simulink model "model21"  (R2021a)
settings: Solver=VariableStepAuto  StartTime=0.0  StopTime=60  RelTol=1e-3
values from neighbouring files (symbols this model uses):
  Ax = 0.8    [model2.m]
  Ay = 0.8    [model2.m]
  Az = 0.4    [model2.m]
  b = 3.59*10^-5    (= 3.59e-05)    [model2.m]
  d = 2.0810*10^-6    (= 2.081e-06)    [model2.m]
  g = 9.81    [model2.m]
  Ix = 0.04439    [model2.m]
  Iy = 0.04439    [model2.m]
  Iz = 0.019    [model2.m]
  J = 0.045    [model2.m]
  l = 0.24    [model2.m]
  m = 0.99285    [model2.m]
undefined symbols (not defined in the file or in its folder): sigbuilder_block
libraries: pid_lib x4
settings Model: Creator=hp  LastModifiedBy=ANUDEEP
settings SolverCC: AlgebraicLoopSolver=TrustRegion
settings DebuggingCC: SFMachineParentedDataDiag=warning

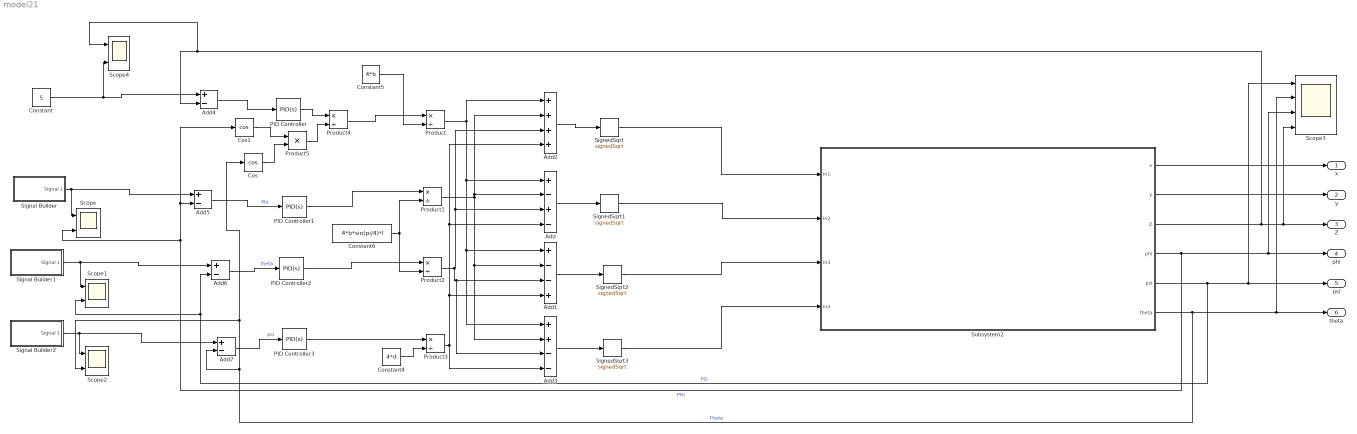
== system model21 ==
  Add : Sum  Inputs=+-+-
  Add1 : Sum  Inputs=+--+
  Add2 : Sum  Inputs=++++
  Add3 : Sum  Inputs=++--
  Add{4..7} (4 alike) : Sum  Inputs=+-
  Constant : Constant  Value=5
  Constant4 : Constant  Value=4*d
  Constant5 : Constant  Value=4*b
  Constant6 : Constant  Value=4*b*sin(pi/4)*l
  Cos : Trigonometry  Operator=cos
  Cos1 : Trigonometry  Operator=cos
  PID Controller : pid_lib/PID Controller  Controller=PID  Form=Parallel  TimeDomain=Continuous-time  UseExternalTs=off  SampleTime=-1  IntegratorMethod=Forward Euler  FilterMethod=Forward Euler  ControllerParametersSource=internal  P=4.3  I=4.5  D=2.05  UseFilter=on  N=100  TunerSelectOption=Transfer Function Based (PID Tuner App)  InitialConditionSource=internal  InitialConditionForIntegrator=0  InitialConditionForFilter=0  DifferentiatorICPrevScaledInput=0  ExternalReset=none  TrackingMode=off  Kt=1  LimitOutput=off  SatLimitsSource=internal  UpperSaturationLimit=inf  LowerSaturationLimit=-inf  LinearizeAsGain=on  AntiWindupMode=none  Kb=1  POutMin=[]  POutMax=[]  IOutMin=[]  IOutMax=[]  DOutMin=[]  DOutMax=[]  NOutMin=[]  NOutMax=[]  SumOutMin=[]  SumOutMax=[]  SaturationOutMin=[]  SaturationOutMax=[]  PParamMin=[]  PParamMax=[]  IParamMin=[]  IParamMax=[]  DParamMin=[]  DParamMax=[]  NParamMin=[]  NParamMax=[]  KbParamMin=[]  KbParamMax=[]  KtParamMin=[]  KtParamMax=[]  KbOutMin=[]  KbOutMax=[]  KtOutMin=[]  KtOutMax=[]  IntegratorOutMin=[]  IntegratorOutMax=[]  FilterOutMin=[]  FilterOutMax=[]  SumI1OutMin=[]  SumI1OutMax=[]  SumI2OutMin=[]  SumI2OutMax=[]  SumI3OutMin=[]  SumI3OutMax=[]  SumI4OutMin=[]  SumI4OutMax=[]  SumDOutMin=[]  SumDOutMax=[]  DifferentiatorOutMin=[]  DifferentiatorOutMax=[]  FilterDiffOutCoefMin=[]  FilterDiffOutCoefMax=[]  ReciprocalOutMin=[]  ReciprocalOutMax=[]  SumDenOutMin=[]  SumDenOutMax=[]  SumNumOutMin=[]  SumNumOutMax=[]  DivideOutMin=[]  DivideOutMax=[]  UdiffTsProdOutMin=[]  UdiffTsProdOutMax=[]  NTsProdOutMin=[]  NTsProdOutMax=[]  UintegralTsProdOutMin=[]  UintegralTsProdOutMax=[]  UngainTsProdOutMin=[]  UngainTsProdOutMax=[]  IntegratorContinuousStateAttributes=''  IntegratorStateMustResolveToSignalObject=off  IntegratorRTWStateStorageClass=Auto  FilterContinuousStateAttributes=''  FilterStateMustResolveToSignalObject=off  FilterRTWStateStorageClass=Auto  ParallelPVariant=InternalParameters  IdealPVariant=Disabled  IVariant=InternalParameters  DVariant=InternalParameters  IntegratorVariant=Continuous  SatVariant=Disabled  AWVariant=Passthrough  PCopyVariant=Disabled  TRVariant=Disabled  FdbkBlocksVariant=Forward  IdealPFdbkVariant=Disabled  SatFdbkVariant=Disabled  DerivativeFilterVariant=ContFilter  NVariant=InternalParameters  NCopyVariant=Disabled  FilterICVariant=InternalICsFilter  IntegratorICVariant=InternalICs  ExternalResetVariant=Disabled  TRSumVariant=Passthrough  SumFdbkVariant=Disabled  SumVariant=Sum_PID  TsampFilterVariant=InternalTs  TsampNgainVariant=Passthrough  TsampIntegralVariant=Passthrough  ExternalSaturationOutDataTypeStr=Inherit: Same as second input
  PID Controller1 : pid_lib/PID Controller  Controller=PID  Form=Parallel  TimeDomain=Continuous-time  UseExternalTs=off  SampleTime=-1  IntegratorMethod=Forward Euler  FilterMethod=Forward Euler  ControllerParametersSource=internal  P=0.262692793721386  I=0.0679116483715347  D=0.252983550233798  UseFilter=on  N=657.62885892053  TunerSelectOption=Transfer Function Based (PID Tuner App)  InitialConditionSource=internal  InitialConditionForIntegrator=0  InitialConditionForFilter=0  DifferentiatorICPrevScaledInput=0  ExternalReset=none  TrackingMode=off  Kt=1  LimitOutput=off  SatLimitsSource=internal  UpperSaturationLimit=inf  LowerSaturationLimit=-inf  LinearizeAsGain=on  AntiWindupMode=none  Kb=1  POutMin=[]  POutMax=[]  IOutMin=[]  IOutMax=[]  DOutMin=[]  DOutMax=[]  NOutMin=[]  NOutMax=[]  SumOutMin=[]  SumOutMax=[]  SaturationOutMin=[]  SaturationOutMax=[]  PParamMin=[]  PParamMax=[]  IParamMin=[]  IParamMax=[]  DParamMin=[]  DParamMax=[]  NParamMin=[]  NParamMax=[]  KbParamMin=[]  KbParamMax=[]  KtParamMin=[]  KtParamMax=[]  KbOutMin=[]  KbOutMax=[]  KtOutMin=[]  KtOutMax=[]  IntegratorOutMin=[]  IntegratorOutMax=[]  FilterOutMin=[]  FilterOutMax=[]  SumI1OutMin=[]  SumI1OutMax=[]  SumI2OutMin=[]  SumI2OutMax=[]  SumI3OutMin=[]  SumI3OutMax=[]  SumI4OutMin=[]  SumI4OutMax=[]  SumDOutMin=[]  SumDOutMax=[]  DifferentiatorOutMin=[]  DifferentiatorOutMax=[]  FilterDiffOutCoefMin=[]  FilterDiffOutCoefMax=[]  ReciprocalOutMin=[]  ReciprocalOutMax=[]  SumDenOutMin=[]  SumDenOutMax=[]  SumNumOutMin=[]  SumNumOutMax=[]  DivideOutMin=[]  DivideOutMax=[]  UdiffTsProdOutMin=[]  UdiffTsProdOutMax=[]  NTsProdOutMin=[]  NTsProdOutMax=[]  UintegralTsProdOutMin=[]  UintegralTsProdOutMax=[]  UngainTsProdOutMin=[]  UngainTsProdOutMax=[]  IntegratorContinuousStateAttributes=''  IntegratorStateMustResolveToSignalObject=off  IntegratorRTWStateStorageClass=Auto  FilterContinuousStateAttributes=''  FilterStateMustResolveToSignalObject=off  FilterRTWStateStorageClass=Auto  ParallelPVariant=InternalParameters  IdealPVariant=Disabled  IVariant=InternalParameters  DVariant=InternalParameters  IntegratorVariant=Continuous  SatVariant=Disabled  AWVariant=Passthrough  PCopyVariant=Disabled  TRVariant=Disabled  FdbkBlocksVariant=Forward  IdealPFdbkVariant=Disabled  SatFdbkVariant=Disabled  DerivativeFilterVariant=ContFilter  NVariant=InternalParameters  NCopyVariant=Disabled  FilterICVariant=InternalICsFilter  IntegratorICVariant=InternalICs  ExternalResetVariant=Disabled  TRSumVariant=Passthrough  SumFdbkVariant=Disabled  SumVariant=Sum_PID  TsampFilterVariant=InternalTs  TsampNgainVariant=Passthrough  TsampIntegralVariant=Passthrough  ExternalSaturationOutDataTypeStr=Inherit: Same as second input
  PID Controller2 : pid_lib/PID Controller  Controller=PID  Form=Parallel  TimeDomain=Continuous-time  UseExternalTs=off  SampleTime=-1  IntegratorMethod=Forward Euler  FilterMethod=Forward Euler  ControllerParametersSource=internal  P=0.314077810197869  I=0.074408762657649  D=0.304896946822323  UseFilter=on  N=790.643788258186  TunerSelectOption=Transfer Function Based (PID Tuner App)  InitialConditionSource=internal  InitialConditionForIntegrator=0  InitialConditionForFilter=0  DifferentiatorICPrevScaledInput=0  ExternalReset=none  TrackingMode=off  Kt=1  LimitOutput=off  SatLimitsSource=internal  UpperSaturationLimit=inf  LowerSaturationLimit=-inf  LinearizeAsGain=on  AntiWindupMode=none  Kb=1  POutMin=[]  POutMax=[]  IOutMin=[]  IOutMax=[]  DOutMin=[]  DOutMax=[]  NOutMin=[]  NOutMax=[]  SumOutMin=[]  SumOutMax=[]  SaturationOutMin=[]  SaturationOutMax=[]  PParamMin=[]  PParamMax=[]  IParamMin=[]  IParamMax=[]  DParamMin=[]  DParamMax=[]  NParamMin=[]  NParamMax=[]  KbParamMin=[]  KbParamMax=[]  KtParamMin=[]  KtParamMax=[]  KbOutMin=[]  KbOutMax=[]  KtOutMin=[]  KtOutMax=[]  IntegratorOutMin=[]  IntegratorOutMax=[]  FilterOutMin=[]  FilterOutMax=[]  SumI1OutMin=[]  SumI1OutMax=[]  SumI2OutMin=[]  SumI2OutMax=[]  SumI3OutMin=[]  SumI3OutMax=[]  SumI4OutMin=[]  SumI4OutMax=[]  SumDOutMin=[]  SumDOutMax=[]  DifferentiatorOutMin=[]  DifferentiatorOutMax=[]  FilterDiffOutCoefMin=[]  FilterDiffOutCoefMax=[]  ReciprocalOutMin=[]  ReciprocalOutMax=[]  SumDenOutMin=[]  SumDenOutMax=[]  SumNumOutMin=[]  SumNumOutMax=[]  DivideOutMin=[]  DivideOutMax=[]  UdiffTsProdOutMin=[]  UdiffTsProdOutMax=[]  NTsProdOutMin=[]  NTsProdOutMax=[]  UintegralTsProdOutMin=[]  UintegralTsProdOutMax=[]  UngainTsProdOutMin=[]  UngainTsProdOutMax=[]  IntegratorContinuousStateAttributes=''  IntegratorStateMustResolveToSignalObject=off  IntegratorRTWStateStorageClass=Auto  FilterContinuousStateAttributes=''  FilterStateMustResolveToSignalObject=off  FilterRTWStateStorageClass=Auto  ParallelPVariant=InternalParameters  IdealPVariant=Disabled  IVariant=InternalParameters  DVariant=InternalParameters  IntegratorVariant=Continuous  SatVariant=Disabled  AWVariant=Passthrough  PCopyVariant=Disabled  TRVariant=Disabled  FdbkBlocksVariant=Forward  IdealPFdbkVariant=Disabled  SatFdbkVariant=Disabled  DerivativeFilterVariant=ContFilter  NVariant=InternalParameters  NCopyVariant=Disabled  FilterICVariant=InternalICsFilter  IntegratorICVariant=InternalICs  ExternalResetVariant=Disabled  TRSumVariant=Passthrough  SumFdbkVariant=Disabled  SumVariant=Sum_PID  TsampFilterVariant=InternalTs  TsampNgainVariant=Passthrough  TsampIntegralVariant=Passthrough  ExternalSaturationOutDataTypeStr=Inherit: Same as second input
  PID Controller3 : pid_lib/PID Controller  Controller=PID  Form=Parallel  TimeDomain=Continuous-time  UseExternalTs=off  SampleTime=-1  IntegratorMethod=Forward Euler  FilterMethod=Forward Euler  ControllerParametersSource=internal  P=0.003528  I=0.0001652  D=0.0185  UseFilter=on  N=5.454  TunerSelectOption=Transfer Function Based (PID Tuner App)  InitialConditionSource=internal  InitialConditionForIntegrator=0  InitialConditionForFilter=0  DifferentiatorICPrevScaledInput=0  ExternalReset=none  TrackingMode=off  Kt=1  LimitOutput=off  SatLimitsSource=internal  UpperSaturationLimit=inf  LowerSaturationLimit=-inf  LinearizeAsGain=on  AntiWindupMode=none  Kb=1  POutMin=[]  POutMax=[]  IOutMin=[]  IOutMax=[]  DOutMin=[]  DOutMax=[]  NOutMin=[]  NOutMax=[]  SumOutMin=[]  SumOutMax=[]  SaturationOutMin=[]  SaturationOutMax=[]  PParamMin=[]  PParamMax=[]  IParamMin=[]  IParamMax=[]  DParamMin=[]  DParamMax=[]  NParamMin=[]  NParamMax=[]  KbParamMin=[]  KbParamMax=[]  KtParamMin=[]  KtParamMax=[]  KbOutMin=[]  KbOutMax=[]  KtOutMin=[]  KtOutMax=[]  IntegratorOutMin=[]  IntegratorOutMax=[]  FilterOutMin=[]  FilterOutMax=[]  SumI1OutMin=[]  SumI1OutMax=[]  SumI2OutMin=[]  SumI2OutMax=[]  SumI3OutMin=[]  SumI3OutMax=[]  SumI4OutMin=[]  SumI4OutMax=[]  SumDOutMin=[]  SumDOutMax=[]  DifferentiatorOutMin=[]  DifferentiatorOutMax=[]  FilterDiffOutCoefMin=[]  FilterDiffOutCoefMax=[]  ReciprocalOutMin=[]  ReciprocalOutMax=[]  SumDenOutMin=[]  SumDenOutMax=[]  SumNumOutMin=[]  SumNumOutMax=[]  DivideOutMin=[]  DivideOutMax=[]  UdiffTsProdOutMin=[]  UdiffTsProdOutMax=[]  NTsProdOutMin=[]  NTsProdOutMax=[]  UintegralTsProdOutMin=[]  UintegralTsProdOutMax=[]  UngainTsProdOutMin=[]  UngainTsProdOutMax=[]  IntegratorContinuousStateAttributes=''  IntegratorStateMustResolveToSignalObject=off  IntegratorRTWStateStorageClass=Auto  FilterContinuousStateAttributes=''  FilterStateMustResolveToSignalObject=off  FilterRTWStateStorageClass=Auto  ParallelPVariant=InternalParameters  IdealPVariant=Disabled  IVariant=InternalParameters  DVariant=InternalParameters  IntegratorVariant=Continuous  SatVariant=Disabled  AWVariant=Passthrough  PCopyVariant=Disabled  TRVariant=Disabled  FdbkBlocksVariant=Forward  IdealPFdbkVariant=Disabled  SatFdbkVariant=Disabled  DerivativeFilterVariant=ContFilter  NVariant=InternalParameters  NCopyVariant=Disabled  FilterICVariant=InternalICsFilter  IntegratorICVariant=InternalICs  ExternalResetVariant=Disabled  TRSumVariant=Passthrough  SumFdbkVariant=Disabled  SumVariant=Sum_PID  TsampFilterVariant=InternalTs  TsampNgainVariant=Passthrough  TsampIntegralVariant=Passthrough  ExternalSaturationOutDataTypeStr=Inherit: Same as second input
  Product{,1..4} (5 alike) : Product  Inputs=*/
  Product5 : Product
  Scope{,1..2,4} (4 alike) : Scope  NumInputPorts=2
  Scope3 : Scope  NumInputPorts=4
  Signal Builder : Subsystem  Tag=STV Subsys  LoadFcn=sigbuilder_block('load');  StartFcn=sigbuilder_block('start');  StopFcn=sigbuilder_block('stop');  ClipboardFcn=sigbuilder_block('clipboard');  mask(Sigbuilder block){tuvar=[0:10]}
      mask help: Simulink:masks:SigbuilderBlock_MD
      mask init:
      | if ~strcmp(get_param(bdroot(gcbh),'SimulationStatus'),'stopped') tuvar = sigbuilder_block('maskInit'); end
      settings: CopyFcn=sigbuilder_block('copy');  DeleteFcn=sigbuilder_block('delete');  ModelCloseFcn=sigbuilder_block('modelClose');  PreSaveFcn=sigbuilder_block('preSave');  PauseFcn=sigbuilder_block('pause');  ContinueFcn=sigbuilder_block('continue');  NameChangeFcn=sigbuilder_block('namechange');  OpenFcn=sigbuilder_block('open',[367.8 129.6 550.8 400.2 ]);  CloseFcn=sigbuilder_block('close');
      mask Display: plot(0, 0, 100, 100,[2, 2, 32, 32, 2], [68, 8, 8, 68, 68],[32, 2], [38, 38], [32, 19, 2],[53, 60, 44], [32, 17, 17, 2],[16, 16, 31, 31]);txt = getActiveGroup(gcbh);text(2, 100, txt,'verticalAlignment', 'top');
  Signal Builder1 : Subsystem  Tag=STV Subsys  LoadFcn=sigbuilder_block('load');  StartFcn=sigbuilder_block('start');  StopFcn=sigbuilder_block('stop');  ClipboardFcn=sigbuilder_block('clipboard');  mask(Sigbuilder block){tuvar=[0:10]}
      mask help: Simulink:masks:SigbuilderBlock_MD
      mask init:
      | if ~strcmp(get_param(bdroot(gcbh),'SimulationStatus'),'stopped') tuvar = sigbuilder_block('maskInit'); end
      settings: CopyFcn=sigbuilder_block('copy');  DeleteFcn=sigbuilder_block('delete');  ModelCloseFcn=sigbuilder_block('modelClose');  PreSaveFcn=sigbuilder_block('preSave');  PauseFcn=sigbuilder_block('pause');  ContinueFcn=sigbuilder_block('continue');  NameChangeFcn=sigbuilder_block('namechange');  OpenFcn=sigbuilder_block('open',[367.8 129.6 550.8 400.2 ]);  CloseFcn=sigbuilder_block('close');
      mask Display: plot(0, 0, 100, 100,[2, 2, 32, 32, 2], [68, 8, 8, 68, 68],[32, 2], [38, 38], [32, 19, 2],[53, 60, 44], [32, 17, 17, 2],[16, 16, 31, 31]);txt = getActiveGroup(gcbh);text(2, 100, txt,'verticalAlignment', 'top');
  Signal Builder2 : Subsystem  Tag=STV Subsys  LoadFcn=sigbuilder_block('load');  StartFcn=sigbuilder_block('start');  StopFcn=sigbuilder_block('stop');  ClipboardFcn=sigbuilder_block('clipboard');  mask(Sigbuilder block){tuvar=[0:10]}
      mask help: Simulink:masks:SigbuilderBlock_MD
      mask init:
      | if ~strcmp(get_param(bdroot(gcbh),'SimulationStatus'),'stopped') tuvar = sigbuilder_block('maskInit'); end
      settings: CopyFcn=sigbuilder_block('copy');  DeleteFcn=sigbuilder_block('delete');  ModelCloseFcn=sigbuilder_block('modelClose');  PreSaveFcn=sigbuilder_block('preSave');  PauseFcn=sigbuilder_block('pause');  ContinueFcn=sigbuilder_block('continue');  NameChangeFcn=sigbuilder_block('namechange');  OpenFcn=sigbuilder_block('open',[345.6 111.6 550.8 400.2 ]);  CloseFcn=sigbuilder_block('close');
      mask Display: plot(0, 0, 100, 100,[2, 2, 32, 32, 2], [68, 8, 8, 68, 68],[32, 2], [38, 38], [32, 19, 2],[53, 60, 44], [32, 17, 17, 2],[16, 16, 31, 31]);txt = getActiveGroup(gcbh);text(2, 100, txt,'verticalAlignment', 'top');
  SignedSqrt{,1..3} (4 alike) : Sqrt  Operator=signedSqrt  OutputSignalType=real  IntermediateResultsDataTypeStr=single  SaturateOnIntegerOverflow=on
  Subsystem2 : Subsystem
  x : Outport
  y : Outport  Port=2
  Z : Outport  Port=3
  phi : Outport  Port=4
  psi : Outport  Port=5
  theta : Outport  Port=6
  wires:
  Product/1 -> Add1/1, Add3/1, Add/1, Add2/1
  Product1/1 -> Add/2, Add2/2, Add1/2, Add3/2
  Product2/1 -> Add3/3, Add1/3, Add/3, Add2/3
  Product3/1 -> Add1/4, Add/4, Add2/4, Add3/4
  Constant4/1 -> Product3/2
  Constant5/1 -> Product/2
  Constant6/1 -> Product1/2, Product2/2
  Product4/1 -> Product/1
  PID Controller/1 -> Product4/1
  Product5/1 -> Product4/2
  Cos/1 -> Product5/2
  Cos1/1 -> Product5/1
  Add4/1 -> PID Controller/1
  PID Controller1/1 -> Product1/1
  PID Controller2/1 -> Product2/1
  PID Controller3/1 -> Product3/1
  Add2/1 -> SignedSqrt/1
  Add/1 -> SignedSqrt1/1
  Add1/1 -> SignedSqrt2/1
  Add3/1 -> SignedSqrt3/1
  Subsystem2/1(x) -> x/1
  Subsystem2/2(y) -> y/1
  Subsystem2/3(Z) -> Scope4/1, Add4/2, Scope3/4, Z/1
  Subsystem2/4(phi) -> Scope/2, Cos1/1, Add5/2, Scope3/3, phi/1  "PHI"
  Subsystem2/5(psi) -> Add6/2, Scope1/2, Scope3/1, psi/1  "PSI"
  Subsystem2/6(theta) -> Add7/2, Scope2/2, Cos/1, Scope3/2, theta/1  "Theta"
  Constant/1 -> Scope4/2, Add4/1
  Signal Builder/1(Signal 1) -> Scope/1, Add5/1
  Signal Builder1/1(Signal 1) -> Scope1/1, Add6/1
  Signal Builder2/1(Signal 1) -> Scope2/1, Add7/1
  Add7/1 -> PID Controller3/1  "psi"
  Add6/1 -> PID Controller2/1  "theta"
  Add5/1 -> PID Controller1/1  "Phi"
  SignedSqrt/1 -> Subsystem2/1(In1)
  SignedSqrt1/1 -> Subsystem2/2(In2)
  SignedSqrt2/1 -> Subsystem2/3(In3)
  SignedSqrt3/1 -> Subsystem2/4(In4)

== system model21/Signal Builder ==
  Demux : Demux  Tag=STV Demux  Outputs=1
      settings: DisplayOption=none
  FromWs : FromWorkspace  Tag=STV FromWs  VariableName=tuvar
      SigBuilderData=|
      | common.afterFinalStr = 'Extrapolate'
      | common.sampleTime = 0
      | dataSet.timeRange = [0 60]
      | dataSet.name = 'Group 1'
      | sbobj.Groups.Name = 'Group 1'
      | sbobj.Groups.Signals.Name = 'Signal 1'
      | sbobj.Groups.Signals.XData = [0 10 10 20 20 50 50 60]
      | sbobj.Groups.Signals.YData = [0 0 0.2 0.2 0 0 0.2 0.2]
      | sbobj.Groups.TimeRange = [0 60]
  Signal 1 : Outport  Tag=STV Outport
  wires:
  Demux/1 -> Signal 1/1
  FromWs/1 -> Demux/1

== system model21/Signal Builder1 ==
  Demux : Demux  Tag=STV Demux  Outputs=1
      settings: DisplayOption=none
  FromWs : FromWorkspace  Tag=STV FromWs  VariableName=tuvar
      SigBuilderData=|
      | common.afterFinalStr = 'Extrapolate'
      | common.sampleTime = 0
      | dataSet.timeRange = [0 60]
      | dataSet.name = 'Group 1'
      | sbobj.Groups.Name = 'Group 1'
      | sbobj.Groups.Signals.Name = 'Signal 1'
      | sbobj.Groups.Signals.XData = [0 30 30 40 40 60]
      | sbobj.Groups.Signals.YData = [0 0 0.2 0.2 0 0]
      | sbobj.Groups.TimeRange = [0 60]
  Signal 1 : Outport  Tag=STV Outport
  wires:
  Demux/1 -> Signal 1/1
  FromWs/1 -> Demux/1

== system model21/Signal Builder2 ==
  Demux : Demux  Tag=STV Demux  Outputs=1
      settings: DisplayOption=none
  FromWs : FromWorkspace  Tag=STV FromWs  VariableName=tuvar
      SigBuilderData=|
      | common.afterFinalStr = 'Extrapolate'
      | common.sampleTime = 0
      | dataSet.timeRange = [0 60]
      | dataSet.name = 'Group 1'
      | sbobj.Groups.Name = 'Group 1'
      | sbobj.Groups.Signals.Name = 'Signal 1'
      | sbobj.Groups.Signals.XData = [0 5 5 10 10 50 60]
      | sbobj.Groups.Signals.YData = [0 0 0.5 0.5 0 0 0]
      | sbobj.Groups.TimeRange = [0 60]
  Signal 1 : Outport  Tag=STV Outport
  wires:
  Demux/1 -> Signal 1/1
  FromWs/1 -> Demux/1

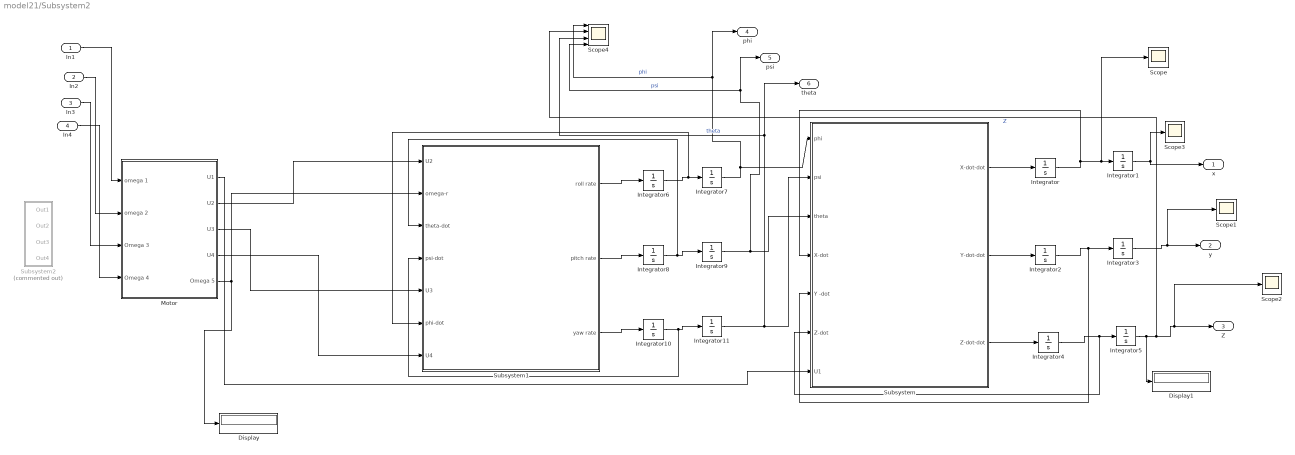
== system model21/Subsystem2 ==
  In1 : Inport
  In2 : Inport  Port=2
  In3 : Inport  Port=3
  In4 : Inport  Port=4
  Display : Display
  Display1 : Display
  Integrator{,1,3..4,6,8,10} (7 alike) : Integrator
  Integrator11 : Integrator  WrapState=on
  Integrator2 : Integrator  LimitOutput=on
  Integrator5 : Integrator  LimitOutput=on  LowerSaturationLimit=0
  Integrator7 : Integrator  WrapState=on
  Integrator9 : Integrator  WrapState=on
  Motor : Subsystem
  Scope{,1..3} (4 alike) : Scope
  Scope4 : Scope  NumInputPorts=4
  Subsystem : Subsystem
  Subsystem1 : Subsystem
  Subsystem2 : Subsystem  Commented=on
  x : Outport
  y : Outport  Port=2
  Z : Outport  Port=3
  phi : Outport  Port=4
  psi : Outport  Port=5
  theta : Outport  Port=6
  wires:
  Integrator9/1 -> psi/1, Scope4/4, Subsystem/3(theta)  "psi"
  Integrator4/1 -> Subsystem/6(Z-dot), Integrator5/1
  Subsystem/3(Z-dot-dot) -> Integrator4/1
  Motor/3(U3) -> Subsystem1/5(U3)
  Motor/2(U2) -> Subsystem1/1(U2)
  Subsystem1/2(pitch rate) -> Integrator8/1
  Integrator6/1 -> Subsystem1/6(phi-dot), Integrator7/1
  Motor/5("Omega 5 ") -> Display/1, Subsystem1/2(omega-r)
  Integrator2/1 -> Subsystem/5(Y -dot), Integrator3/1
  Integrator1/1 -> x/1, Scope3/1
  Integrator5/1 -> Display1/1, Z/1, Scope2/1, Scope4/2  "Z"
  Integrator/1 -> Subsystem/4(X-dot), Scope/1, Integrator1/1
  Subsystem/2(Y-dot-dot) -> Integrator2/1
  Subsystem1/1(roll rate) -> Integrator6/1
  Motor/1(U1) -> Subsystem/7(U1)
  Integrator3/1 -> y/1, Scope1/1
  Integrator7/1 -> phi/1, Scope4/1, Subsystem/1(phi)  "phi"
  Motor/4(U4) -> Subsystem1/7(U4)
  Integrator8/1 -> Subsystem1/3(theta-dot), Integrator9/1
  Integrator10/1 -> Subsystem1/4(psi-dot), Integrator11/1
  Subsystem/1(X-dot-dot) -> Integrator/1
  Subsystem1/3(yaw rate) -> Integrator10/1
  Integrator11/1 -> theta/1, Scope4/3, Subsystem/2(psi)  "theta"
  In4/1 -> Motor/4(Omega 4)
  In3/1 -> Motor/3(Omega 3)
  In2/1 -> Motor/2(omega 2)
  In1/1 -> Motor/1(omega 1)

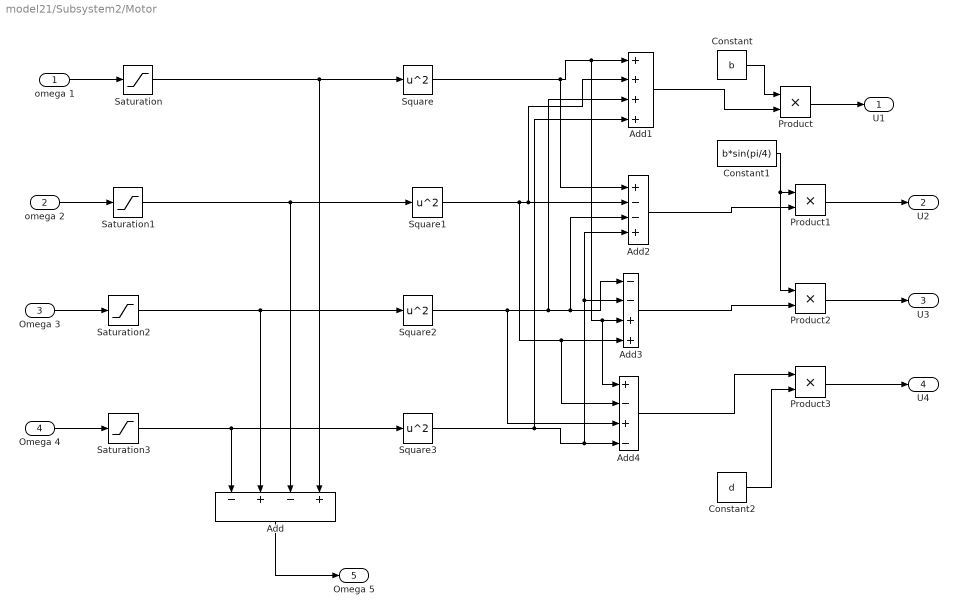
== system model21/Subsystem2/Motor ==
  omega 1 : Inport
  omega 2 : Inport  Port=2
  Omega 3 : Inport  Port=3
  Omega 4 : Inport  Port=4
  Add : Sum  Inputs=-+-+
  Add1 : Sum  Inputs=++++
  Add2 : Sum  Inputs=+--+
  Add3 : Sum  Inputs=--++
  Add4 : Sum  Inputs=+-+-
  Constant : Constant  Value=b
  Constant1 : Constant  Value=b*sin(pi/4)
  Constant2 : Constant  Value=d
  Product{,1..3} (4 alike) : Product
  Saturation{,1..3} (4 alike) : Saturate  UpperLimit=10000  LowerLimit=-10000
  Square{,1..3} (4 alike) : Math  Operator=square  SaturateOnIntegerOverflow=on
  U1 : Outport
  U2 : Outport  Port=2
  U3 : Outport  Port=3
  U4 : Outport  Port=4
  "Omega 5 " : Outport  Port=5
  wires:
  Add4/1 -> Product3/1
  Square3/1 -> Add1/4, Add3/2, Add2/4, Add4/4
  Square1/1 -> Add4/2, Add3/4, Add1/2, Add2/2
  Square/1 -> Add2/1, Add3/3, Add4/1, Add1/1
  Constant1/1 -> Product1/1, Product2/1
  Square2/1 -> Add4/3, Add1/3, Add2/3, Add3/1
  omega 1/1 -> Saturation/1
  Saturation1/1 -> Square1/1, Add/3
  Add3/1 -> Product2/2
  Product3/1 -> U4/1
  Constant2/1 -> Product3/2
  Saturation3/1 -> Add/1, Square3/1
  omega 2/1 -> Saturation1/1
  Saturation2/1 -> Square2/1, Add/2
  Add2/1 -> Product1/2
  Product1/1 -> U2/1
  Add/1 -> "Omega 5 "/1
  Constant/1 -> Product/1
  Saturation/1 -> Square/1, Add/4
  Product2/1 -> U3/1
  Omega 4/1 -> Saturation3/1
  Product/1 -> U1/1
  Add1/1 -> Product/2
  Omega 3/1 -> Saturation2/1

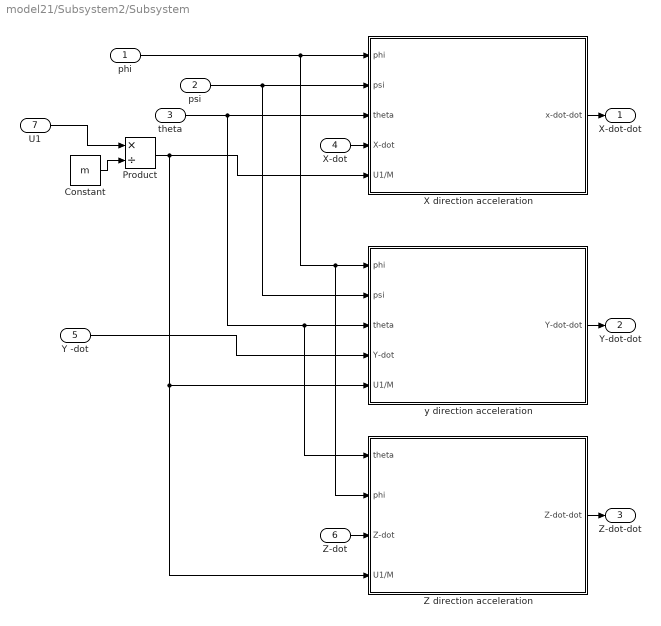
== system model21/Subsystem2/Subsystem ==
  phi : Inport
  psi : Inport  Port=2
  theta : Inport  Port=3
  X-dot : Inport  Port=4
  Y -dot : Inport  Port=5
  Z-dot : Inport  Port=6
  U1 : Inport  Port=7
  " y direction acceleration" : Subsystem
  Constant : Constant  Value=m
  Product : Product  Inputs=*/
  X direction acceleration : Subsystem
  Z direction acceleration : Subsystem
  X-dot-dot : Outport
  Y-dot-dot : Outport  Port=2
  Z-dot-dot : Outport  Port=3
  wires:
  psi/1 -> " y direction acceleration"/2(psi), X direction acceleration/2(psi)
  X direction acceleration/1(x-dot-dot) -> X-dot-dot/1
  Product/1 -> X direction acceleration/5(U1/M), Z direction acceleration/4(U1/M), " y direction acceleration"/5(U1/M)
  Z-dot/1 -> Z direction acceleration/3(Z-dot)
  X-dot/1 -> X direction acceleration/4(X-dot)
  theta/1 -> Z direction acceleration/1(theta), " y direction acceleration"/3(theta), X direction acceleration/3(theta)
  " y direction acceleration"/1(Y-dot-dot) -> Y-dot-dot/1
  phi/1 -> X direction acceleration/1(phi), Z direction acceleration/2(phi), " y direction acceleration"/1(phi)
  Y -dot/1 -> " y direction acceleration"/4(Y-dot)
  Z direction acceleration/1(Z-dot-dot) -> Z-dot-dot/1
  Constant/1 -> Product/2
  U1/1 -> Product/1

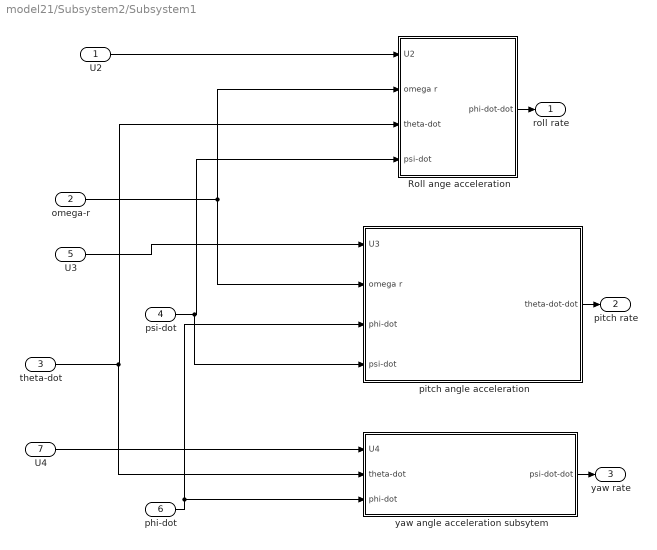
== system model21/Subsystem2/Subsystem1 ==
  U2 : Inport
  omega-r : Inport  Port=2
  theta-dot : Inport  Port=3
  psi-dot : Inport  Port=4
  U3 : Inport  Port=5
  phi-dot : Inport  Port=6
  U4 : Inport  Port=7
  Roll ange acceleration : Subsystem
  pitch angle acceleration : Subsystem
  "yaw angle acceleration subsytem " : Subsystem
  roll rate : Outport
  pitch rate : Outport  Port=2
  yaw rate : Outport  Port=3
  wires:
  theta-dot/1 -> "yaw angle acceleration subsytem "/2(theta-dot), Roll ange acceleration/3(theta-dot)
  U4/1 -> "yaw angle acceleration subsytem "/1(U4)
  Roll ange acceleration/1(phi-dot-dot) -> roll rate/1
  U2/1 -> Roll ange acceleration/1(U2)
  "yaw angle acceleration subsytem "/1(psi-dot-dot) -> yaw rate/1
  U3/1 -> pitch angle acceleration/1(U3)
  psi-dot/1 -> pitch angle acceleration/4(psi-dot), Roll ange acceleration/4(psi-dot)
  pitch angle acceleration/1(theta-dot-dot) -> pitch rate/1
  omega-r/1 -> Roll ange acceleration/2(omega r), pitch angle acceleration/2(omega r)
  phi-dot/1 -> "yaw angle acceleration subsytem "/3(phi-dot), pitch angle acceleration/3(phi-dot)

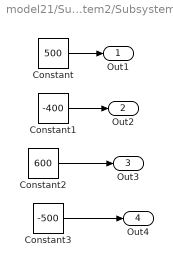
== system model21/Subsystem2/Subsystem2 ==
  Constant : Constant  Value=500
  Constant1 : Constant  Value=-400
  Constant2 : Constant  Value=600
  Constant3 : Constant  Value=-500
  Out1 : Outport
  Out2 : Outport  Port=2
  Out3 : Outport  Port=3
  Out4 : Outport  Port=4
  wires:
  Constant3/1 -> Out4/1
  Constant1/1 -> Out2/1
  Constant2/1 -> Out3/1
  Constant/1 -> Out1/1

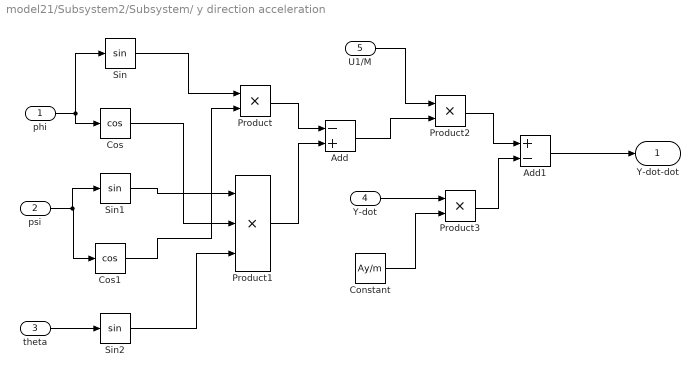
== system model21/Subsystem2/Subsystem/ y direction acceleration ==
  phi : Inport
  psi : Inport  Port=2
  theta : Inport  Port=3
  Y-dot : Inport  Port=4
  U1/M : Inport  Port=5
  Add : Sum  Inputs=-+
  Add1 : Sum  Inputs=+-
  Constant : Constant  Value=Ay/m
  Cos : Trigonometry  Operator=cos
  Cos1 : Trigonometry  Operator=cos
  Product : Product
  Product1 : Product  Inputs=3
  Product2 : Product
  Product3 : Product
  Sin : Trigonometry
  Sin1 : Trigonometry
  Sin2 : Trigonometry
  Y-dot-dot : Outport
  wires:
  theta/1 -> Sin2/1
  Product/1 -> Add/1
  phi/1 -> Sin/1, Cos/1
  Sin/1 -> Product/1
  Y-dot/1 -> Product3/1
  Cos1/1 -> Product/2
  Add1/1 -> Y-dot-dot/1
  U1/M/1 -> Product2/1
  Sin2/1 -> Product1/3
  Constant/1 -> Product3/2
  Product2/1 -> Add1/1
  Cos/1 -> Product1/2
  Add/1 -> Product2/2
  psi/1 -> Sin1/1, Cos1/1
  Product1/1 -> Add/2
  Product3/1 -> Add1/2
  Sin1/1 -> Product1/1

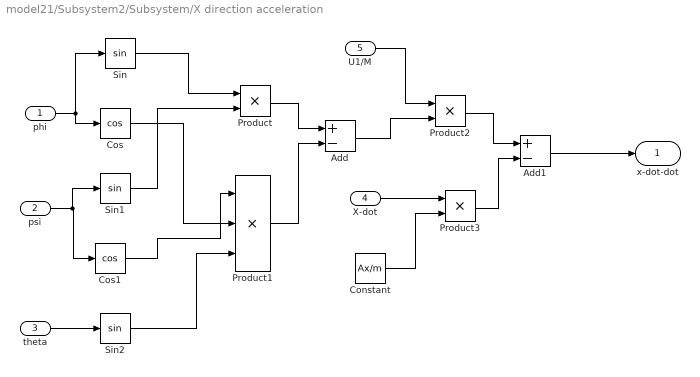
== system model21/Subsystem2/Subsystem/X direction acceleration ==
  phi : Inport
  psi : Inport  Port=2
  theta : Inport  Port=3
  X-dot : Inport  Port=4
  U1/M : Inport  Port=5
  Add : Sum  Inputs=+-
  Add1 : Sum  Inputs=+-
  Constant : Constant  Value=Ax/m
  Cos : Trigonometry  Operator=cos
  Cos1 : Trigonometry  Operator=cos
  Product : Product
  Product1 : Product  Inputs=3
  Product2 : Product
  Product3 : Product
  Sin : Trigonometry
  Sin1 : Trigonometry
  Sin2 : Trigonometry
  x-dot-dot : Outport
  wires:
  Add/1 -> Product2/2
  Product/1 -> Add/1
  Product1/1 -> Add/2
  U1/M/1 -> Product2/1
  Sin/1 -> Product/1
  phi/1 -> Sin/1, Cos/1
  Cos/1 -> Product1/2
  Sin1/1 -> Product/2
  Cos1/1 -> Product1/1
  Sin2/1 -> Product1/3
  theta/1 -> Sin2/1
  psi/1 -> Sin1/1, Cos1/1
  Product3/1 -> Add1/2
  Product2/1 -> Add1/1
  X-dot/1 -> Product3/1
  Constant/1 -> Product3/2
  Add1/1 -> x-dot-dot/1

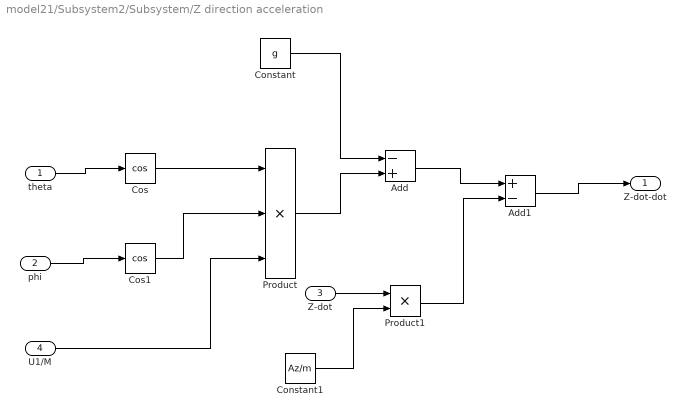
== system model21/Subsystem2/Subsystem/Z direction acceleration ==
  theta : Inport
  phi : Inport  Port=2
  Z-dot : Inport  Port=3
  U1/M : Inport  Port=4
  Add : Sum  Inputs=-+
  Add1 : Sum  Inputs=+-
  Constant : Constant  Value=g
  Constant1 : Constant  Value=Az/m
  Cos : Trigonometry  Operator=cos
  Cos1 : Trigonometry  Operator=cos
  Product : Product  Inputs=3
  Product1 : Product
  Z-dot-dot : Outport
  wires:
  theta/1 -> Cos/1
  phi/1 -> Cos1/1
  U1/M/1 -> Product/3
  Cos1/1 -> Product/2
  Cos/1 -> Product/1
  Constant/1 -> Add/1
  Product/1 -> Add/2
  Constant1/1 -> Product1/2
  Z-dot/1 -> Product1/1
  Add1/1 -> Z-dot-dot/1
  Add/1 -> Add1/1
  Product1/1 -> Add1/2

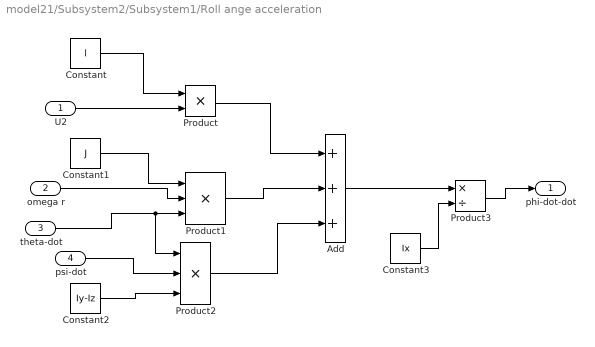
== system model21/Subsystem2/Subsystem1/Roll ange acceleration ==
  U2 : Inport
  omega r : Inport  Port=2
  theta-dot : Inport  Port=3
  psi-dot : Inport  Port=4
  Add : Sum  Inputs=+++
  Constant : Constant  Value=l
  Constant1 : Constant  Value=J
  Constant2 : Constant  Value=Iy-Iz
  Constant3 : Constant  Value=Ix
  Product : Product
  Product1 : Product  Inputs=3
  Product2 : Product  Inputs=3
  Product3 : Product  Inputs=*/
  phi-dot-dot : Outport
  wires:
  U2/1 -> Product/2
  Constant/1 -> Product/1
  Product/1 -> Add/1
  Product1/1 -> Add/2
  Constant1/1 -> Product1/1
  omega r/1 -> Product1/2
  theta-dot/1 -> Product2/1, Product1/3
  psi-dot/1 -> Product2/2
  Constant2/1 -> Product2/3
  Product2/1 -> Add/3
  Add/1 -> Product3/1
  Constant3/1 -> Product3/2
  Product3/1 -> phi-dot-dot/1

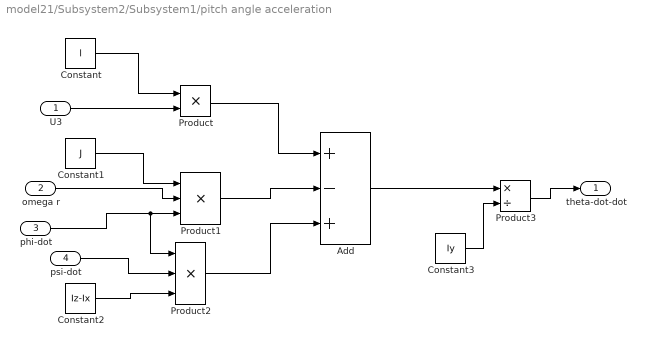
== system model21/Subsystem2/Subsystem1/pitch angle acceleration ==
  U3 : Inport
  omega r : Inport  Port=2
  phi-dot : Inport  Port=3
  psi-dot : Inport  Port=4
  Add : Sum  Inputs=+-+
  Constant : Constant  Value=l
  Constant1 : Constant  Value=J
  Constant2 : Constant  Value=Iz-Ix
  Constant3 : Constant  Value=Iy
  Product : Product
  Product1 : Product  Inputs=3
  Product2 : Product  Inputs=3
  Product3 : Product  Inputs=*/
  theta-dot-dot : Outport
  wires:
  Constant1/1 -> Product1/1
  Constant2/1 -> Product2/3
  Product2/1 -> Add/3
  Product1/1 -> Add/2
  Product3/1 -> theta-dot-dot/1
  Constant3/1 -> Product3/2
  Constant/1 -> Product/1
  U3/1 -> Product/2
  phi-dot/1 -> Product2/1, Product1/3
  Product/1 -> Add/1
  Add/1 -> Product3/1
  omega r/1 -> Product1/2
  psi-dot/1 -> Product2/2

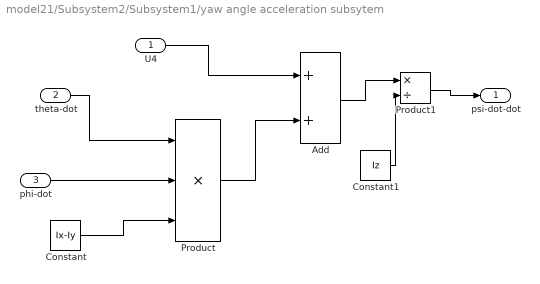
== system model21/Subsystem2/Subsystem1/yaw angle acceleration subsytem  ==
  U4 : Inport
  theta-dot : Inport  Port=2
  phi-dot : Inport  Port=3
  Add : Sum
  Constant : Constant  Value=Ix-Iy
  Constant1 : Constant  Value=Iz
  Product : Product  Inputs=3
  Product1 : Product  Inputs=*/
  psi-dot-dot : Outport
  wires:
  Product/1 -> Add/2
  U4/1 -> Add/1
  phi-dot/1 -> Product/2
  theta-dot/1 -> Product/1
  Constant/1 -> Product/3
  Add/1 -> Product1/1
  Constant1/1 -> Product1/2
  Product1/1 -> psi-dot-dot/1
